simulink model "Waehrungsmodelle"  (R2014a)
settings: Solver=ode1  StartTime=0.0  StopTime=100  FixedStep=1  MaxStep=1  MinStep=1  RelTol=1e-3
(part 12 of 18)

== system Waehrungsmodelle/Währungssystem1/Notenbank ==
  Gesamtkredite : Inport
  Arbeitslosenquote : Inport  Port=2
  Wirtschaftswachtsum : Inport  Port=3
  Inflation : Inport  Port=4
  MATLAB Function : MATLAB Function  TreatAsAtomicUnit=on
  Leitzinssatz der Notenbank : Outport
  Mindestreservesatz von der Notenbank : Outport  Port=2
  Maximale Geldmenge von der Notenbank : Outport  Port=3
  wires:
  MATLAB Function/2(MindestreservesatzOut) -> Mindestreservesatz von der Notenbank/1
  MATLAB Function/3(MaximaleNotenbankGeldmengeOut) -> Maximale Geldmenge von der Notenbank/1
  MATLAB Function/1(LeitzinsOut) -> Leitzinssatz der Notenbank/1
  Wirtschaftswachtsum/1 -> MATLAB Function/4(Wirtschaftswachtsum)
  Arbeitslosenquote/1 -> MATLAB Function/2(Arbeitslosenquote)
  Gesamtkredite/1 -> MATLAB Function/1(Gesamtkredite)
  Inflation/1 -> MATLAB Function/3(Inflation)

== system Waehrungsmodelle/Währungssystem1/Populationsmodell ==
  note: Geburten
  Umweltqualität : Inport
  Dienstleistungsqualität : Inport  Port=2
  Güterangebotsqualität bei vorhandem Einkommen : Inport  Port=3
  Ausgleichsfaktor : Constant  Value=0.3
  Dienstleistungs- multiplikator : Sum
  Divide1 : Product  Inputs=*/
  Divide2 : Product  Inputs=*/
  Divide3 : Product  Inputs=*/
  Erwachsene : Sum  Inputs=+--
  Fertilitätsmultiplikator : Product  Inputs=4
  Fertilitätsrate pro Frau : Constant  Value=3/40
  Frauenanteil pro Erwachsene : Constant  Value=0.5
  Güterangebotsqualitäts- multiplikator : Sum
  Jahre der Altersklasse : Constant  Value=15
  Jahre der Altersklasse1 : Constant  Value=10
  Jahre der Altersklasse2 : Constant  Value=40
  Kinder : Sum  Inputs=+--
  Lebensqualitätsfaktor : Product  Inputs=/
  Product{,1..3} (4 alike) : Product  Inputs=3
  Schüler / Studenten : Sum  Inputs=+--
  Start Erwachsene: 55 : Integrator  InitialCondition=55
  Start Kinder: 13 : Integrator  InitialCondition=13
  Start Schüler: 11 : Integrator  InitialCondition=11
  Sterblichkeitsrate Kinder : Constant  Value=0.003
  Sterblichkeitsrate1 : Constant  Value=0.002
  Sterblichkeitsrate2 : Constant  Value=0.004
  Umwelt- multiplikator : Sum
  Erwerbsfähige : Outport
  wires:
  Product/1 -> Kinder/1
  Jahre der Altersklasse2/1 -> Divide3/2
  Jahre der Altersklasse/1 -> Divide1/2
  Divide1/1 -> Schüler / Studenten/1, Kinder/3
  Sterblichkeitsrate1/1 -> Product1/2
  Sterblichkeitsrate Kinder/1 -> Product2/2
  Divide2/1 -> Schüler / Studenten/3, Erwachsene/1
  Start Schüler: 11/1 -> Product1/3, Divide2/1
  Jahre der Altersklasse1/1 -> Divide2/2
  Sterblichkeitsrate2/1 -> Product3/2
  Start Erwachsene: 55/1 -> Erwerbsfähige/1, Product3/3, Divide3/1, Product/1
  Erwachsene/1 -> Start Erwachsene: 55/1
  Kinder/1 -> Start Kinder: 13/1
  Start Kinder: 13/1 -> Product2/3, Divide1/1
  Schüler / Studenten/1 -> Start Schüler: 11/1
  Ausgleichsfaktor/1 -> Umwelt- multiplikator/2, Güterangebotsqualitäts- multiplikator/1, Dienstleistungs- multiplikator/1
  Fertilitätsmultiplikator/1 -> Product/3
  Umweltqualität/1 -> Umwelt- multiplikator/1
  Dienstleistungs- multiplikator/1 -> Lebensqualitätsfaktor/1, Fertilitätsmultiplikator/4
  Fertilitätsrate pro Frau/1 -> Fertilitätsmultiplikator/1
  Umwelt- multiplikator/1 -> Fertilitätsmultiplikator/2
  Dienstleistungsqualität/1 -> Dienstleistungs- multiplikator/2
  Product2/1 -> Kinder/2
  Product1/1 -> Schüler / Studenten/2
  Divide3/1 -> Erwachsene/3
  Product3/1 -> Erwachsene/2
  Lebensqualitätsfaktor/1 -> Product3/1, Product1/1, Product2/1
  Güterangebotsqualität bei vorhandem Einkommen/1 -> Güterangebotsqualitäts- multiplikator/2
  Güterangebotsqualitäts- multiplikator/1 -> Fertilitätsmultiplikator/3
  Frauenanteil pro Erwachsene/1 -> Product/2

== system Waehrungsmodelle/Währungssystem1/Staat ==
  Kreditvergabe : Inport
  Kreditrückzahlung : Inport  Port=2
  Finanzbedarf Arbeitslosigkeit : Inport  Port=3
  Dienstleistungsqualität : Inport  Port=4
  Steuern Bank : Inport  Port=5
  Steuern Unternehmen : Inport  Port=6
  Rohstoffabgabe : Inport  Port=7
  Umweltqualität : Inport  Port=8
  MATLAB Function : MATLAB Function  TreatAsAtomicUnit=on
  Kreditbedarf : Outport
  Finanzierung Öffentlicher Dienstleistungen : Outport  Port=2
  Geldbestand Staat : Outport  Port=3
  Steuersatz : Outport  Port=4
  Ressourcen Steuer : Outport  Port=5
  wires:
  Steuern Unternehmen/1 -> MATLAB Function/6(SteuernUnternehmen)
  Dienstleistungsqualität/1 -> MATLAB Function/4(Dienstleistungsqualitaet)
  MATLAB Function/4(SteuersatzOut) -> Steuersatz/1
  MATLAB Function/2(FinanzierungOeffentlicheDienstleistungen) -> Finanzierung Öffentlicher Dienstleistungen/1
  Finanzbedarf Arbeitslosigkeit/1 -> MATLAB Function/3(FinanzbedarfArbeitslosigkeit)
  MATLAB Function/3(GeldbestandStaat) -> Geldbestand Staat/1
  Kreditrückzahlung/1 -> MATLAB Function/2(Kreditrueckzahlung)
  MATLAB Function/1(Kreditbedarf) -> Kreditbedarf/1
  Steuern Bank/1 -> MATLAB Function/5(SteuernBanken)
  Kreditvergabe/1 -> MATLAB Function/1(KreditvergabeNeuStaat)
  MATLAB Function/5(RessourcenAbgabesatzOut) -> Ressourcen Steuer/1
  Rohstoffabgabe/1 -> MATLAB Function/7(Rohstoffabgabe)
  Umweltqualität/1 -> MATLAB Function/8(Umweltqualitaet)

== system Waehrungsmodelle/Währungssystem1/Umwelt ==
  Ressourcenbedarf : Inport
  Umwelt : MATLAB Function  TreatAsAtomicUnit=on
  abgebaute Ressourcen : Outport
  verhandene Ressourcen : Outport  Port=2
  Umweltqualität : Outport  Port=3
  wires:
  Umwelt/3(Umweltqualitaet) -> Umweltqualität/1
  Umwelt/2(VorhandeneRessourcenOut) -> verhandene Ressourcen/1
  Umwelt/1(AbgebauteRessourcen) -> abgebaute Ressourcen/1
  Ressourcenbedarf/1 -> Umwelt/1(Ressourcenbedarf)

== system Waehrungsmodelle/Währungssystem1/Unternehmen ==
  Erwerbsfähige : Inport
  Neue Kreditvergabe der Unternehmen : Inport  Port=2
  Kreditrückzahlung der Unternehmen : Inport  Port=3
  Rohstoffe : Inport  Port=4
  Güterkonsum Inland : Inport  Port=5
  Güterkonsum Ausland : Inport  Port=6
  RessourcenAbgabe Steuersatz : Inport  Port=7
  Kreditzinssatz Inland : Inport  Port=8
  Kreditzinssatz Ausland : Inport  Port=9
  Steuersatz : Inport  Port=10
  Neue Kreditvergabe der Unternehmen Ausland : Inport  Port=11
  Kreditrückzahlung der Unternehmen Ausland : Inport  Port=12
  MATLAB Function : MATLAB Function  TreatAsAtomicUnit=on
  Inflation : Outport
  Rohstoffbedarf : Outport  Port=2
  Arbeitsplätze der Unternehmen : Outport  Port=3
  Güterangebot Inland : Outport  Port=4
  Arbeitslohn : Outport  Port=5
  zukünftiger Arbeitsdarf der Unternehmen : Outport  Port=6
  Güterpreis : Outport  Port=7
  Steuern von Unternehmen : Outport  Port=8
  Rohstoffabgabe : Outport  Port=9
  Kreditbedarf Inland : Outport  Port=10
  Kreditbedarf Ausland : Outport  Port=11
  Technischer Fortschritt Rationalität : Outport  Port=12
  Technischer Fortschritt Ressourcen : Outport  Port=13
  Wirtschaftswachstum : Outport  Port=14
  Güterangebot Ausland : Outport  Port=15
  wires:
  MATLAB Function/8(SteuernUnternehmen) -> Steuern von Unternehmen/1
  MATLAB Function/7(GueterpreisOut) -> Güterpreis/1
  Neue Kreditvergabe der Unternehmen/1 -> MATLAB Function/2(NeueKreditvergabeUnternehmen)
  Kreditrückzahlung der Unternehmen/1 -> MATLAB Function/3(KreditrueckzahlungUnternehmen)
  MATLAB Function/6(BenoetigterArbeitsbedarfUnternehmen) -> zukünftiger Arbeitsdarf der Unternehmen/1
  MATLAB Function/4(GueterangebotInland) -> Güterangebot Inland/1
  MATLAB Function/5(ArbeitslohnOut) -> Arbeitslohn/1
  MATLAB Function/2(Rohstoffbedarf) -> Rohstoffbedarf/1
  MATLAB Function/1(Inflation) -> Inflation/1
  Erwerbsfähige/1 -> MATLAB Function/1(Erwerbsfaehige)
  MATLAB Function/3(ArbeitsplaetzeUnternehmen) -> Arbeitsplätze der Unternehmen/1
  Rohstoffe/1 -> MATLAB Function/4(Rohstoffe)
  Güterkonsum Inland/1 -> MATLAB Function/5(GueterkonsumInland)
  MATLAB Function/9(RessourcenAbgabeSteuer) -> Rohstoffabgabe/1
  MATLAB Function/11(KreditbedarfAusland) -> Kreditbedarf Ausland/1
  MATLAB Function/12(TechnischeVerbesserungRationalitaetOut) -> Technischer Fortschritt Rationalität/1
  MATLAB Function/13(TechnischeVerbesserungRessourcenOut) -> Technischer Fortschritt Ressourcen/1
  Güterkonsum Ausland/1 -> MATLAB Function/6(GueterkonsumAusland)
  RessourcenAbgabe Steuersatz/1 -> MATLAB Function/7(RessourcenAbgabeSteuersatz)
  Kreditzinssatz Inland/1 -> MATLAB Function/8(KreditZinssatzInland)
  Kreditzinssatz Ausland/1 -> MATLAB Function/9(KreditZinssatzAusland)
  Steuersatz/1 -> MATLAB Function/10(Steuersatz)
  MATLAB Function/10(KreditbedarfInland) -> Kreditbedarf Inland/1
  MATLAB Function/14(Wirtschaftswachstum) -> Wirtschaftswachstum/1
  MATLAB Function/15(GueterangebotAusland) -> Güterangebot Ausland/1
  Neue Kreditvergabe der Unternehmen Ausland/1 -> MATLAB Function/11(NeueKreditvergabeUnternehmenAusland)
  Kreditrückzahlung der Unternehmen Ausland/1 -> MATLAB Function/12(KreditrueckzahlungUnternehmenAusland)

== system Waehrungsmodelle/Währungssystem1/Wechselkursberechnung ==
  Güterpreis Ausland : Inport
  Güterkonsum im Inland von Gütern vom Ausland : Inport  Port=2
  Güterkonsum im Ausland von Gütern im Inland : Inport  Port=3
  MATLAB Function : MATLAB Function  TreatAsAtomicUnit=on
  Güterpreis Ausland in Eigenwährung : Outport
  Wechselkursfaktor : Outport  Port=2
  Gesamter Güterkonsum im Ausland von Gütern im Inland : Outport  Port=3
  Gesamter Güterkonsum im Inland von Gütern vom Ausland : Outport  Port=4
  wires:
  Güterpreis Ausland/1 -> MATLAB Function/1(GueterpreisAusland)
  Güterkonsum im Inland von Gütern vom Ausland/1 -> MATLAB Function/2(GueterKonsumImInlandVomAusland)
  Güterkonsum im Ausland von Gütern im Inland/1 -> MATLAB Function/3(GueterKonsumImAuslandVomInland)
  MATLAB Function/1(GueterpreisAuslandInEigenwaehrung) -> Güterpreis Ausland in Eigenwährung/1
  MATLAB Function/2(Wechselkursfaktor) -> Wechselkursfaktor/1
  MATLAB Function/3(GesamterGueterKonsumImAuslandVomInlandOut) -> Gesamter Güterkonsum im Ausland von Gütern im Inland/1
  MATLAB Function/4(GesamterGueterKonsumImInlandVomAuslandOut) -> Gesamter Güterkonsum im Inland von Gütern vom Ausland/1

== system Waehrungsmodelle/Währungssystem1/Öffentliche Dienstleistungen ==
  Finanzierung : Inport
  Erwerbsfähige : Inport  Port=2
  Arbeitslohn : Inport  Port=3
  MATLAB Function : MATLAB Function  TreatAsAtomicUnit=on
  Arbeitsplätze Dienstleistung : Outport
  Dienstleistungsqualität : Outport  Port=2
  wires:
  Arbeitslohn/1 -> MATLAB Function/3(Arbeitslohn)
  Erwerbsfähige/1 -> MATLAB Function/2(Erwerbsfaehige)
  Finanzierung/1 -> MATLAB Function/1(Finanzierung)
  MATLAB Function/1(ArbeitsplaetzeDienstleistung) -> Arbeitsplätze Dienstleistung/1
  MATLAB Function/2(Dienstleistungsqualitaet) -> Dienstleistungsqualität/1

== system Waehrungsmodelle/Währungssystem2/Banken ==
  Einlangenänderung der Haushalte : Inport
  Kreditbedarf der Haushalte : Inport  Port=2
  Kreditbedarf der Unternehmen : Inport  Port=3
  Kreditbedarf der Haushalte im Ausland : Inport  Port=4
  Kreditbedarf der Unternehmen im Ausland : Inport  Port=5
  Kreditbedarf des Staates : Inport  Port=6
  Steuersatz : Inport  Port=7
  Leitzins der Notenbank : Inport  Port=8
  Mindestreservesatz der Notenbank : Inport  Port=9
  Maximale Geldmenge der Notebank : Inport  Port=10
  MATLAB Function : MATLAB Function  TreatAsAtomicUnit=on
  Kontostand der Haushalte : Outport
  Kredite der Haushalte : Outport  Port=2
  Kredite der Unternehmen : Outport  Port=3
  Kredite des Staates : Outport  Port=4
  Neue Kreditvergabe Haushalte : Outport  Port=5
  Neue Kreditvergabe Unternehmen : Outport  Port=6
  Neue Kreditvergabe Staat : Outport  Port=7
  Bankgewinn nach Steuern : Outport  Port=8
  Banksteuern : Outport  Port=9
  Bankkontostand : Outport  Port=10
  Bankenzinssatz : Outport  Port=11
  Kreditrückzahlung Staat : Outport  Port=12
  Kreditrückzahlung Haushalte : Outport  Port=13
  Kreditrückzahlung Unternehmen : Outport  Port=14
  Kredite der Unternehmen im Ausland : Outport  Port=15
  Kreditrückzahlung der Unternehmen im Ausland : Outport  Port=16
  Kreditvergabe der Unternehmen im Ausland : Outport  Port=17
  Kredite der Haushalte im Ausland : Outport  Port=18
  Kreditrückzahlung der Haushalte im Ausland : Outport  Port=19
  Kreditvergabe der Haushalte im Ausland : Outport  Port=20
  wires:
  MATLAB Function/1(KontoHaushalteOut) -> Kontostand der Haushalte/1
  MATLAB Function/2(KrediteHaushalteOut) -> Kredite der Haushalte/1
  MATLAB Function/3(KrediteUnternehmenOut) -> Kredite der Unternehmen/1
  MATLAB Function/4(KrediteStaatOut) -> Kredite des Staates/1
  MATLAB Function/5(KreditvergabeHaushalte) -> Neue Kreditvergabe Haushalte/1
  MATLAB Function/6(KreditvergabeUnternehmen) -> Neue Kreditvergabe Unternehmen/1
  MATLAB Function/7(KreditvergabeStaat) -> Neue Kreditvergabe Staat/1
  MATLAB Function/11(BankgewinnNachSteuern) -> Bankgewinn nach Steuern/1
  MATLAB Function/10(KreditrueckzahlungStaat) -> Kreditrückzahlung Staat/1
  MATLAB Function/9(KreditrueckzahlungUnternehmen) -> Kreditrückzahlung Unternehmen/1
  MATLAB Function/8(KreditrueckzahlungHaushalte) -> Kreditrückzahlung Haushalte/1
  MATLAB Function/14(Bankenzinssatz) -> Bankenzinssatz/1
  MATLAB Function/13(BankKontostand) -> Bankkontostand/1
  MATLAB Function/12(BankenSteuern) -> Banksteuern/1
  MATLAB Function/15(KrediteUnternehmenAuslandOut) -> Kredite der Unternehmen im Ausland/1
  MATLAB Function/16(KreditrueckzahlungUnternehmenAusland) -> Kreditrückzahlung der Unternehmen im Ausland/1
  MATLAB Function/17(KreditvergabeUnternehmenAusland) -> Kreditvergabe der Unternehmen im Ausland/1
  MATLAB Function/18(KrediteHaushalteAuslandOut) -> Kredite der Haushalte im Ausland/1
  MATLAB Function/20(KreditvergabeHaushalteAusland) -> Kreditvergabe der Haushalte im Ausland/1
  MATLAB Function/19(KreditrueckzahlungHaushalteAusland) -> Kreditrückzahlung der Haushalte im Ausland/1
  Einlangenänderung der Haushalte/1 -> MATLAB Function/1(EinlagenAenderungHaushalte)
  Kreditbedarf der Haushalte/1 -> MATLAB Function/2(KreditbedarfHaushalte)
  Kreditbedarf der Unternehmen/1 -> MATLAB Function/3(KreditbedarfUnternehmen)
  Kreditbedarf der Haushalte im Ausland/1 -> MATLAB Function/4(KreditbedarfHaushalteAusland)
  Kreditbedarf der Unternehmen im Ausland/1 -> MATLAB Function/5(KreditbedarfUnternehmenAusland)
  Kreditbedarf des Staates/1 -> MATLAB Function/6(KreditbedarfStaat)
  Steuersatz/1 -> MATLAB Function/7(Steuersatz)
  Leitzins der Notenbank/1 -> MATLAB Function/8(Leitzins)
  Mindestreservesatz der Notenbank/1 -> MATLAB Function/9(Mindestreservesatz)
  Maximale Geldmenge der Notebank/1 -> MATLAB Function/10(MaximaleNotenbankGeldmenge)

== system Waehrungsmodelle/Währungssystem2/Haushalte ==
  Erwerbsfähige : Inport
  Arbeitsplätze Dienstleistungen : Inport  Port=2
  Güterangebot Inland : Inport  Port=3
  Arbeitslohn : Inport  Port=4
  Güterpreis Inland : Inport  Port=5
  Neue Kreditvergabe Inland : Inport  Port=6
  Arbeitsplätze Unternehmen : Inport  Port=7
  Kreditrückzahlung Ausland : Inport  Port=8
  Güterpreis Ausland : Inport  Port=9
  Neue Kreditvergabe Ausland : Inport  Port=10
  Kreditrückzahlung Inland : Inport  Port=11
  Güterangebot Ausland : Inport  Port=12
  Kreditzinssatz Inland : Inport  Port=13
  Kreditzinssatz Ausland : Inport  Port=14
  MATLAB Function : MATLAB Function  TreatAsAtomicUnit=on
  Güterkonsum Inland : Outport
  Finanzbedarf Arbeitslosigkeit : Outport  Port=2
  Spareinlagen : Outport  Port=3
  Kreditbedarf Inland : Outport  Port=4
  Arbeiter Unternehmen : Outport  Port=5
  Gütervorrat der Haushalte : Outport  Port=6
  Güterangebotsqualität : Outport  Port=7
  Arbeitslosenquote : Outport  Port=8
  Güterkonsum Ausland : Outport  Port=9
  Kreditbedarf Ausland : Outport  Port=10
  wires:
  Arbeitslohn/1 -> MATLAB Function/7(Arbeitslohn)
  Erwerbsfähige/1 -> MATLAB Function/1(Erwerbsfaehige)
  Arbeitsplätze Dienstleistungen/1 -> MATLAB Function/2(ArbeitsplaetzeDienstleistungen)
  Güterangebot Inland/1 -> MATLAB Function/6(GueterAngebotInland)
  Güterpreis Inland/1 -> MATLAB Function/8(GueterpreisInland)
  MATLAB Function/1(GueterkonsumInland) -> Güterkonsum Inland/1
  MATLAB Function/2(FinanzierungArbeitslosigkeit) -> Finanzbedarf Arbeitslosigkeit/1
  MATLAB Function/4(KreditbedarfInland) -> Kreditbedarf Inland/1
  MATLAB Function/5(ArbeiterUnternehmen) -> Arbeiter Unternehmen/1
  MATLAB Function/3(Spareinlagen) -> Spareinlagen/1
  Neue Kreditvergabe Inland/1 -> MATLAB Function/4(NeueKreditvergabeInland)
  Arbeitsplätze Unternehmen/1 -> MATLAB Function/3(ArbeitsplaetzeUnternehmen)
  MATLAB Function/6(GueterVorratHaushalte) -> Gütervorrat der Haushalte/1
  MATLAB Function/7(GueterangebotsqualitaetOut) -> Güterangebotsqualität/1
  Kreditrückzahlung Ausland/1 -> MATLAB Function/5(KreditrueckzahlungInland)
  MATLAB Function/8(Arbeitslosenquote) -> Arbeitslosenquote/1
  MATLAB Function/9(GueterkonsumAusland) -> Güterkonsum Ausland/1
  MATLAB Function/10(KreditbedarfAusland) -> Kreditbedarf Ausland/1
  Güterpreis Ausland/1 -> MATLAB Function/9(GueterpreisAusland)
  Neue Kreditvergabe Ausland/1 -> MATLAB Function/10(NeueKreditvergabeAusland)
  Kreditrückzahlung Inland/1 -> MATLAB Function/11(KreditrueckzahlungAusland)
  Güterangebot Ausland/1 -> MATLAB Function/12(GueterAngebotAusland)
  Kreditzinssatz Inland/1 -> MATLAB Function/13(KreditZinssatzInland)
  Kreditzinssatz Ausland/1 -> MATLAB Function/14(KreditZinssatzAusland)

== system Waehrungsmodelle/Währungssystem2/Notenbank ==
  Gesamtkredite : Inport
  Arbeitslosenquote : Inport  Port=2
  Wirtschaftswachtsum : Inport  Port=3
  Inflation : Inport  Port=4
  MATLAB Function : MATLAB Function  TreatAsAtomicUnit=on
  Leitzinssatz der Notenbank : Outport
  Mindestreservesatz von der Notenbank : Outport  Port=2
  Maximale Geldmenge von der Notenbank : Outport  Port=3
  wires:
  MATLAB Function/2(MindestreservesatzOut) -> Mindestreservesatz von der Notenbank/1
  MATLAB Function/3(MaximaleNotenbankGeldmengeOut) -> Maximale Geldmenge von der Notenbank/1
  MATLAB Function/1(LeitzinsOut) -> Leitzinssatz der Notenbank/1
  Wirtschaftswachtsum/1 -> MATLAB Function/4(Wirtschaftswachtsum)
  Arbeitslosenquote/1 -> MATLAB Function/2(Arbeitslosenquote)
  Gesamtkredite/1 -> MATLAB Function/1(Gesamtkredite)
  Inflation/1 -> MATLAB Function/3(Inflation)

== system Waehrungsmodelle/Währungssystem2/Populationsmodell ==
  note: Geburten
  Umweltqualität : Inport
  Dienstleistungsqualität : Inport  Port=2
  Güterangebotsqualität bei vorhandem Einkommen : Inport  Port=3
  Ausgleichsfaktor : Constant  Value=0.3
  Dienstleistungs- multiplikator : Sum
  Divide1 : Product  Inputs=*/
  Divide2 : Product  Inputs=*/
  Divide3 : Product  Inputs=*/
  Erwachsene : Sum  Inputs=+--
  Fertilitätsmultiplikator : Product  Inputs=4
  Fertilitätsrate pro Frau : Constant  Value=3/40
  Frauenanteil pro Erwachsene : Constant  Value=0.5
  Güterangebotsqualitäts- multiplikator : Sum
  Jahre der Altersklasse : Constant  Value=15
  Jahre der Altersklasse1 : Constant  Value=10
  Jahre der Altersklasse2 : Constant  Value=40
  Kinder : Sum  Inputs=+--
  Lebensqualitätsfaktor : Product  Inputs=/
  Product{,1..3} (4 alike) : Product  Inputs=3
  Schüler / Studenten : Sum  Inputs=+--
  Start Erwachsene: 55 : Integrator  InitialCondition=55
  Start Kinder: 13 : Integrator  InitialCondition=13
  Start Schüler: 11 : Integrator  InitialCondition=11
  Sterblichkeitsrate Kinder : Constant  Value=0.003
  Sterblichkeitsrate1 : Constant  Value=0.002
  Sterblichkeitsrate2 : Constant  Value=0.004
  Umwelt- multiplikator : Sum
  Erwerbsfähige : Outport
  wires:
  Product/1 -> Kinder/1
  Jahre der Altersklasse2/1 -> Divide3/2
  Jahre der Altersklasse/1 -> Divide1/2
  Divide1/1 -> Schüler / Studenten/1, Kinder/3
  Sterblichkeitsrate1/1 -> Product1/2
  Sterblichkeitsrate Kinder/1 -> Product2/2
  Divide2/1 -> Schüler / Studenten/3, Erwachsene/1
  Start Schüler: 11/1 -> Product1/3, Divide2/1
  Jahre der Altersklasse1/1 -> Divide2/2
  Sterblichkeitsrate2/1 -> Product3/2
  Start Erwachsene: 55/1 -> Erwerbsfähige/1, Product3/3, Divide3/1, Product/1
  Erwachsene/1 -> Start Erwachsene: 55/1
  Kinder/1 -> Start Kinder: 13/1
  Start Kinder: 13/1 -> Product2/3, Divide1/1
  Schüler / Studenten/1 -> Start Schüler: 11/1
  Ausgleichsfaktor/1 -> Umwelt- multiplikator/2, Güterangebotsqualitäts- multiplikator/1, Dienstleistungs- multiplikator/1
  Fertilitätsmultiplikator/1 -> Product/3
  Umweltqualität/1 -> Umwelt- multiplikator/1
  Dienstleistungs- multiplikator/1 -> Lebensqualitätsfaktor/1, Fertilitätsmultiplikator/4
  Fertilitätsrate pro Frau/1 -> Fertilitätsmultiplikator/1
  Umwelt- multiplikator/1 -> Fertilitätsmultiplikator/2
  Dienstleistungsqualität/1 -> Dienstleistungs- multiplikator/2
  Product2/1 -> Kinder/2
  Product1/1 -> Schüler / Studenten/2
  Divide3/1 -> Erwachsene/3
  Product3/1 -> Erwachsene/2
  Lebensqualitätsfaktor/1 -> Product3/1, Product1/1, Product2/1
  Güterangebotsqualität bei vorhandem Einkommen/1 -> Güterangebotsqualitäts- multiplikator/2
  Güterangebotsqualitäts- multiplikator/1 -> Fertilitätsmultiplikator/3
  Frauenanteil pro Erwachsene/1 -> Product/2

== system Waehrungsmodelle/Währungssystem2/Staat ==
  Kreditvergabe : Inport
  Kreditrückzahlung : Inport  Port=2
  Finanzbedarf Arbeitslosigkeit : Inport  Port=3
  Dienstleistungsqualität : Inport  Port=4
  Steuern Bank : Inport  Port=5
  Steuern Unternehmen : Inport  Port=6
  Rohstoffabgabe : Inport  Port=7
  Umweltqualität : Inport  Port=8
  MATLAB Function : MATLAB Function  TreatAsAtomicUnit=on
  Kreditbedarf : Outport
  Finanzierung Öffentlicher Dienstleistungen : Outport  Port=2
  Geldbestand Staat : Outport  Port=3
  Steuersatz : Outport  Port=4
  Ressourcen Steuer : Outport  Port=5
  wires:
  Steuern Unternehmen/1 -> MATLAB Function/6(SteuernUnternehmen)
  Dienstleistungsqualität/1 -> MATLAB Function/4(Dienstleistungsqualitaet)
  MATLAB Function/4(SteuersatzOut) -> Steuersatz/1
  MATLAB Function/2(FinanzierungOeffentlicheDienstleistungen) -> Finanzierung Öffentlicher Dienstleistungen/1
  Finanzbedarf Arbeitslosigkeit/1 -> MATLAB Function/3(FinanzbedarfArbeitslosigkeit)
  MATLAB Function/3(GeldbestandStaat) -> Geldbestand Staat/1
  Kreditrückzahlung/1 -> MATLAB Function/2(Kreditrueckzahlung)
  MATLAB Function/1(Kreditbedarf) -> Kreditbedarf/1
  Steuern Bank/1 -> MATLAB Function/5(SteuernBanken)
  Kreditvergabe/1 -> MATLAB Function/1(KreditvergabeNeuStaat)
  MATLAB Function/5(RessourcenAbgabesatzOut) -> Ressourcen Steuer/1
  Rohstoffabgabe/1 -> MATLAB Function/7(Rohstoffabgabe)
  Umweltqualität/1 -> MATLAB Function/8(Umweltqualitaet)

== system Waehrungsmodelle/Währungssystem2/Umwelt ==
  Ressourcenbedarf : Inport
  Umwelt : MATLAB Function  TreatAsAtomicUnit=on
  abgebaute Ressourcen : Outport
  verhandene Ressourcen : Outport  Port=2
  Umweltqualität : Outport  Port=3
  wires:
  Umwelt/3(Umweltqualitaet) -> Umweltqualität/1
  Umwelt/2(VorhandeneRessourcenOut) -> verhandene Ressourcen/1
  Umwelt/1(AbgebauteRessourcen) -> abgebaute Ressourcen/1
  Ressourcenbedarf/1 -> Umwelt/1(Ressourcenbedarf)

== system Waehrungsmodelle/Währungssystem2/Unternehmen ==
  Erwerbsfähige : Inport
  Neue Kreditvergabe der Unternehmen : Inport  Port=2
  Kreditrückzahlung der Unternehmen : Inport  Port=3
  Rohstoffe : Inport  Port=4
  Güterkonsum Inland : Inport  Port=5
  Güterkonsum Ausland : Inport  Port=6
  RessourcenAbgabe Steuersatz : Inport  Port=7
  Kreditzinssatz Inland : Inport  Port=8
  Kreditzinssatz Ausland : Inport  Port=9
  Steuersatz : Inport  Port=10
  Neue Kreditvergabe der Unternehmen Ausland : Inport  Port=11
  Kreditrückzahlung der Unternehmen Ausland : Inport  Port=12
  MATLAB Function : MATLAB Function  TreatAsAtomicUnit=on
  Inflation : Outport
  Rohstoffbedarf : Outport  Port=2
  Arbeitsplätze der Unternehmen : Outport  Port=3
  Güterangebot Inland : Outport  Port=4
  Arbeitslohn : Outport  Port=5
  zukünftiger Arbeitsdarf der Unternehmen : Outport  Port=6
  Güterpreis : Outport  Port=7
  Steuern von Unternehmen : Outport  Port=8
  Rohstoffabgabe : Outport  Port=9
  Kreditbedarf Inland : Outport  Port=10
  Kreditbedarf Ausland : Outport  Port=11
  Technischer Fortschritt Rationalität : Outport  Port=12
  Technischer Fortschritt Ressourcen : Outport  Port=13
  Wirtschaftswachstum : Outport  Port=14
  Güterangebot Ausland : Outport  Port=15
  wires:
  MATLAB Function/8(SteuernUnternehmen) -> Steuern von Unternehmen/1
  MATLAB Function/7(GueterpreisOut) -> Güterpreis/1
  Neue Kreditvergabe der Unternehmen/1 -> MATLAB Function/2(NeueKreditvergabeUnternehmen)
  Kreditrückzahlung der Unternehmen/1 -> MATLAB Function/3(KreditrueckzahlungUnternehmen)
  MATLAB Function/6(BenoetigterArbeitsbedarfUnternehmen) -> zukünftiger Arbeitsdarf der Unternehmen/1
  MATLAB Function/4(GueterangebotInland) -> Güterangebot Inland/1
  MATLAB Function/5(ArbeitslohnOut) -> Arbeitslohn/1
  MATLAB Function/2(Rohstoffbedarf) -> Rohstoffbedarf/1
  MATLAB Function/1(Inflation) -> Inflation/1
  Erwerbsfähige/1 -> MATLAB Function/1(Erwerbsfaehige)
  MATLAB Function/3(ArbeitsplaetzeUnternehmen) -> Arbeitsplätze der Unternehmen/1
  Rohstoffe/1 -> MATLAB Function/4(Rohstoffe)
  Güterkonsum Inland/1 -> MATLAB Function/5(GueterkonsumInland)
  MATLAB Function/9(RessourcenAbgabeSteuer) -> Rohstoffabgabe/1
  MATLAB Function/11(KreditbedarfAusland) -> Kreditbedarf Ausland/1
  MATLAB Function/12(TechnischeVerbesserungRationalitaetOut) -> Technischer Fortschritt Rationalität/1
  MATLAB Function/13(TechnischeVerbesserungRessourcenOut) -> Technischer Fortschritt Ressourcen/1
  Güterkonsum Ausland/1 -> MATLAB Function/6(GueterkonsumAusland)
  RessourcenAbgabe Steuersatz/1 -> MATLAB Function/7(RessourcenAbgabeSteuersatz)
  Kreditzinssatz Inland/1 -> MATLAB Function/8(KreditZinssatzInland)
  Kreditzinssatz Ausland/1 -> MATLAB Function/9(KreditZinssatzAusland)
  Steuersatz/1 -> MATLAB Function/10(Steuersatz)
  MATLAB Function/10(KreditbedarfInland) -> Kreditbedarf Inland/1
  MATLAB Function/14(Wirtschaftswachstum) -> Wirtschaftswachstum/1
  MATLAB Function/15(GueterangebotAusland) -> Güterangebot Ausland/1
  Neue Kreditvergabe der Unternehmen Ausland/1 -> MATLAB Function/11(NeueKreditvergabeUnternehmenAusland)
  Kreditrückzahlung der Unternehmen Ausland/1 -> MATLAB Function/12(KreditrueckzahlungUnternehmenAusland)

== system Waehrungsmodelle/Währungssystem2/Wechselkursberechnung ==
  Güterpreis Ausland : Inport
  Güterkonsum im Inland von Gütern vom Ausland : Inport  Port=2
  Güterkonsum im Ausland von Gütern im Inland : Inport  Port=3
  MATLAB Function : MATLAB Function  TreatAsAtomicUnit=on
  Güterpreis Ausland in Eigenwährung : Outport
  Wechselkursfaktor : Outport  Port=2
  Gesamter Güterkonsum im Ausland von Gütern im Inland : Outport  Port=3
  Gesamter Güterkonsum im Inland von Gütern vom Ausland : Outport  Port=4
  wires:
  Güterpreis Ausland/1 -> MATLAB Function/1(GueterpreisAusland)
  Güterkonsum im Inland von Gütern vom Ausland/1 -> MATLAB Function/2(GueterKonsumImInlandVomAusland)
  Güterkonsum im Ausland von Gütern im Inland/1 -> MATLAB Function/3(GueterKonsumImAuslandVomInland)
  MATLAB Function/1(GueterpreisAuslandInEigenwaehrung) -> Güterpreis Ausland in Eigenwährung/1
  MATLAB Function/2(Wechselkursfaktor) -> Wechselkursfaktor/1
  MATLAB Function/3(GesamterGueterKonsumImAuslandVomInlandOut) -> Gesamter Güterkonsum im Ausland von Gütern im Inland/1
  MATLAB Function/4(GesamterGueterKonsumImInlandVomAuslandOut) -> Gesamter Güterkonsum im Inland von Gütern vom Ausland/1

== system Waehrungsmodelle/Währungssystem2/Öffentliche Dienstleistungen ==
  Finanzierung : Inport
  Erwerbsfähige : Inport  Port=2
  Arbeitslohn : Inport  Port=3
  MATLAB Function : MATLAB Function  TreatAsAtomicUnit=on
  Arbeitsplätze Dienstleistung : Outport
  Dienstleistungsqualität : Outport  Port=2
  wires:
  Arbeitslohn/1 -> MATLAB Function/3(Arbeitslohn)
  Erwerbsfähige/1 -> MATLAB Function/2(Erwerbsfaehige)
  Finanzierung/1 -> MATLAB Function/1(Finanzierung)
  MATLAB Function/1(ArbeitsplaetzeDienstleistung) -> Arbeitsplätze Dienstleistung/1
  MATLAB Function/2(Dienstleistungsqualitaet) -> Dienstleistungsqualität/1

== system Waehrungsmodelle/Währungssystem3/Banken ==
  Einlangenänderung der Haushalte : Inport
  Kreditbedarf der Haushalte : Inport  Port=2
  Kreditbedarf der Unternehmen : Inport  Port=3
  Kreditbedarf der Haushalte im Ausland : Inport  Port=4
  Kreditbedarf der Unternehmen im Ausland : Inport  Port=5
  Kreditbedarf des Staates : Inport  Port=6
  Steuersatz : Inport  Port=7
  Leitzins der Notenbank : Inport  Port=8
  Mindestreservesatz der Notenbank : Inport  Port=9
  Maximale Geldmenge der Notebank : Inport  Port=10
  MATLAB Function : MATLAB Function  TreatAsAtomicUnit=on
  Kontostand der Haushalte : Outport
  Kredite der Haushalte : Outport  Port=2
  Kredite der Unternehmen : Outport  Port=3
  Kredite des Staates : Outport  Port=4
  Neue Kreditvergabe Haushalte : Outport  Port=5
  Neue Kreditvergabe Unternehmen : Outport  Port=6
  Neue Kreditvergabe Staat : Outport  Port=7
  Bankgewinn nach Steuern : Outport  Port=8
  Banksteuern : Outport  Port=9
  Bankkontostand : Outport  Port=10
  Bankenzinssatz : Outport  Port=11
  Kreditrückzahlung Staat : Outport  Port=12
  Kreditrückzahlung Haushalte : Outport  Port=13
  Kreditrückzahlung Unternehmen : Outport  Port=14
  Kredite der Unternehmen im Ausland : Outport  Port=15
  Kreditrückzahlung der Unternehmen im Ausland : Outport  Port=16
  Kreditvergabe der Unternehmen im Ausland : Outport  Port=17
  Kredite der Haushalte im Ausland : Outport  Port=18
  Kreditrückzahlung der Haushalte im Ausland : Outport  Port=19
  Kreditvergabe der Haushalte im Ausland : Outport  Port=20
  wires:
  MATLAB Function/1(KontoHaushalteOut) -> Kontostand der Haushalte/1
  MATLAB Function/2(KrediteHaushalteOut) -> Kredite der Haushalte/1
  MATLAB Function/3(KrediteUnternehmenOut) -> Kredite der Unternehmen/1
  MATLAB Function/4(KrediteStaatOut) -> Kredite des Staates/1
  MATLAB Function/5(KreditvergabeHaushalte) -> Neue Kreditvergabe Haushalte/1
  MATLAB Function/6(KreditvergabeUnternehmen) -> Neue Kreditvergabe Unternehmen/1
  MATLAB Function/7(KreditvergabeStaat) -> Neue Kreditvergabe Staat/1
  MATLAB Function/11(BankgewinnNachSteuern) -> Bankgewinn nach Steuern/1
  MATLAB Function/10(KreditrueckzahlungStaat) -> Kreditrückzahlung Staat/1
  MATLAB Function/9(KreditrueckzahlungUnternehmen) -> Kreditrückzahlung Unternehmen/1
  MATLAB Function/8(KreditrueckzahlungHaushalte) -> Kreditrückzahlung Haushalte/1
  MATLAB Function/14(Bankenzinssatz) -> Bankenzinssatz/1
  MATLAB Function/13(BankKontostand) -> Bankkontostand/1
  MATLAB Function/12(BankenSteuern) -> Banksteuern/1
  MATLAB Function/15(KrediteUnternehmenAuslandOut) -> Kredite der Unternehmen im Ausland/1
  MATLAB Function/16(KreditrueckzahlungUnternehmenAusland) -> Kreditrückzahlung der Unternehmen im Ausland/1
  MATLAB Function/17(KreditvergabeUnternehmenAusland) -> Kreditvergabe der Unternehmen im Ausland/1
  MATLAB Function/18(KrediteHaushalteAuslandOut) -> Kredite der Haushalte im Ausland/1
  MATLAB Function/20(KreditvergabeHaushalteAusland) -> Kreditvergabe der Haushalte im Ausland/1
  MATLAB Function/19(KreditrueckzahlungHaushalteAusland) -> Kreditrückzahlung der Haushalte im Ausland/1
  Einlangenänderung der Haushalte/1 -> MATLAB Function/1(EinlagenAenderungHaushalte)
  Kreditbedarf der Haushalte/1 -> MATLAB Function/2(KreditbedarfHaushalte)
  Kreditbedarf der Unternehmen/1 -> MATLAB Function/3(KreditbedarfUnternehmen)
  Kreditbedarf der Haushalte im Ausland/1 -> MATLAB Function/4(KreditbedarfHaushalteAusland)
  Kreditbedarf der Unternehmen im Ausland/1 -> MATLAB Function/5(KreditbedarfUnternehmenAusland)
  Kreditbedarf des Staates/1 -> MATLAB Function/6(KreditbedarfStaat)
  Steuersatz/1 -> MATLAB Function/7(Steuersatz)
  Leitzins der Notenbank/1 -> MATLAB Function/8(Leitzins)
  Mindestreservesatz der Notenbank/1 -> MATLAB Function/9(Mindestreservesatz)
  Maximale Geldmenge der Notebank/1 -> MATLAB Function/10(MaximaleNotenbankGeldmenge)

== system Waehrungsmodelle/Währungssystem3/Haushalte ==
  Erwerbsfähige : Inport
  Arbeitsplätze Dienstleistungen : Inport  Port=2
  Güterangebot Inland : Inport  Port=3
  Arbeitslohn : Inport  Port=4
  Güterpreis Inland : Inport  Port=5
  Neue Kreditvergabe Inland : Inport  Port=6
  Arbeitsplätze Unternehmen : Inport  Port=7
  Kreditrückzahlung Ausland : Inport  Port=8
  Güterpreis Ausland : Inport  Port=9
  Neue Kreditvergabe Ausland : Inport  Port=10
  Kreditrückzahlung Inland : Inport  Port=11
  Güterangebot Ausland : Inport  Port=12
  Kreditzinssatz Inland : Inport  Port=13
  Kreditzinssatz Ausland : Inport  Port=14
  MATLAB Function : MATLAB Function  TreatAsAtomicUnit=on
  Güterkonsum Inland : Outport
  Finanzbedarf Arbeitslosigkeit : Outport  Port=2
  Spareinlagen : Outport  Port=3
  Kreditbedarf Inland : Outport  Port=4
  Arbeiter Unternehmen : Outport  Port=5
  Gütervorrat der Haushalte : Outport  Port=6
  Güterangebotsqualität : Outport  Port=7
  Arbeitslosenquote : Outport  Port=8
  Güterkonsum Ausland : Outport  Port=9
  Kreditbedarf Ausland : Outport  Port=10
  wires:
  Arbeitslohn/1 -> MATLAB Function/7(Arbeitslohn)
  Erwerbsfähige/1 -> MATLAB Function/1(Erwerbsfaehige)
  Arbeitsplätze Dienstleistungen/1 -> MATLAB Function/2(ArbeitsplaetzeDienstleistungen)
  Güterangebot Inland/1 -> MATLAB Function/6(GueterAngebotInland)
  Güterpreis Inland/1 -> MATLAB Function/8(GueterpreisInland)
  MATLAB Function/1(GueterkonsumInland) -> Güterkonsum Inland/1
  MATLAB Function/2(FinanzierungArbeitslosigkeit) -> Finanzbedarf Arbeitslosigkeit/1
  MATLAB Function/4(KreditbedarfInland) -> Kreditbedarf Inland/1
  MATLAB Function/5(ArbeiterUnternehmen) -> Arbeiter Unternehmen/1
  MATLAB Function/3(Spareinlagen) -> Spareinlagen/1
  Neue Kreditvergabe Inland/1 -> MATLAB Function/4(NeueKreditvergabeInland)
  Arbeitsplätze Unternehmen/1 -> MATLAB Function/3(ArbeitsplaetzeUnternehmen)
  MATLAB Function/6(GueterVorratHaushalte) -> Gütervorrat der Haushalte/1
  MATLAB Function/7(GueterangebotsqualitaetOut) -> Güterangebotsqualität/1
  Kreditrückzahlung Ausland/1 -> MATLAB Function/5(KreditrueckzahlungInland)
  MATLAB Function/8(Arbeitslosenquote) -> Arbeitslosenquote/1
  MATLAB Function/9(GueterkonsumAusland) -> Güterkonsum Ausland/1
  MATLAB Function/10(KreditbedarfAusland) -> Kreditbedarf Ausland/1
  Güterpreis Ausland/1 -> MATLAB Function/9(GueterpreisAusland)
  Neue Kreditvergabe Ausland/1 -> MATLAB Function/10(NeueKreditvergabeAusland)
  Kreditrückzahlung Inland/1 -> MATLAB Function/11(KreditrueckzahlungAusland)
  Güterangebot Ausland/1 -> MATLAB Function/12(GueterAngebotAusland)
  Kreditzinssatz Inland/1 -> MATLAB Function/13(KreditZinssatzInland)
  Kreditzinssatz Ausland/1 -> MATLAB Function/14(KreditZinssatzAusland)

== system Waehrungsmodelle/Währungssystem3/Notenbank ==
  Gesamtkredite : Inport
  Arbeitslosenquote : Inport  Port=2
  Wirtschaftswachtsum : Inport  Port=3
  Inflation : Inport  Port=4
  MATLAB Function : MATLAB Function  TreatAsAtomicUnit=on
  Leitzinssatz der Notenbank : Outport
  Mindestreservesatz von der Notenbank : Outport  Port=2
  Maximale Geldmenge von der Notenbank : Outport  Port=3
  wires:
  MATLAB Function/2(MindestreservesatzOut) -> Mindestreservesatz von der Notenbank/1
  MATLAB Function/3(MaximaleNotenbankGeldmengeOut) -> Maximale Geldmenge von der Notenbank/1
  MATLAB Function/1(LeitzinsOut) -> Leitzinssatz der Notenbank/1
  Wirtschaftswachtsum/1 -> MATLAB Function/4(Wirtschaftswachtsum)
  Arbeitslosenquote/1 -> MATLAB Function/2(Arbeitslosenquote)
  Gesamtkredite/1 -> MATLAB Function/1(Gesamtkredite)
  Inflation/1 -> MATLAB Function/3(Inflation)

== system Waehrungsmodelle/Währungssystem3/Populationsmodell ==
  note: Geburten
  Umweltqualität : Inport
  Dienstleistungsqualität : Inport  Port=2
  Güterangebotsqualität bei vorhandem Einkommen : Inport  Port=3
  Ausgleichsfaktor : Constant  Value=0.3
  Dienstleistungs- multiplikator : Sum
  Divide1 : Product  Inputs=*/
  Divide2 : Product  Inputs=*/
  Divide3 : Product  Inputs=*/
  Erwachsene : Sum  Inputs=+--
  Fertilitätsmultiplikator : Product  Inputs=4
  Fertilitätsrate pro Frau : Constant  Value=3/40
  Frauenanteil pro Erwachsene : Constant  Value=0.5
  Güterangebotsqualitäts- multiplikator : Sum
  Jahre der Altersklasse : Constant  Value=15
  Jahre der Altersklasse1 : Constant  Value=10
  Jahre der Altersklasse2 : Constant  Value=40
  Kinder : Sum  Inputs=+--
  Lebensqualitätsfaktor : Product  Inputs=/
  Product{,1..3} (4 alike) : Product  Inputs=3
  Schüler / Studenten : Sum  Inputs=+--
  Start Erwachsene: 55 : Integrator  InitialCondition=55
  Start Kinder: 13 : Integrator  InitialCondition=13
  Start Schüler: 11 : Integrator  InitialCondition=11
  Sterblichkeitsrate Kinder : Constant  Value=0.003
  Sterblichkeitsrate1 : Constant  Value=0.002
  Sterblichkeitsrate2 : Constant  Value=0.004
  Umwelt- multiplikator : Sum
  Erwerbsfähige : Outport
  wires:
  Product/1 -> Kinder/1
  Jahre der Altersklasse2/1 -> Divide3/2
  Jahre der Altersklasse/1 -> Divide1/2
  Divide1/1 -> Schüler / Studenten/1, Kinder/3
  Sterblichkeitsrate1/1 -> Product1/2
  Sterblichkeitsrate Kinder/1 -> Product2/2
  Divide2/1 -> Schüler / Studenten/3, Erwachsene/1
  Start Schüler: 11/1 -> Product1/3, Divide2/1
  Jahre der Altersklasse1/1 -> Divide2/2
  Sterblichkeitsrate2/1 -> Product3/2
  Start Erwachsene: 55/1 -> Erwerbsfähige/1, Product3/3, Divide3/1, Product/1
  Erwachsene/1 -> Start Erwachsene: 55/1
  Kinder/1 -> Start Kinder: 13/1
  Start Kinder: 13/1 -> Product2/3, Divide1/1
  Schüler / Studenten/1 -> Start Schüler: 11/1
  Ausgleichsfaktor/1 -> Umwelt- multiplikator/2, Güterangebotsqualitäts- multiplikator/1, Dienstleistungs- multiplikator/1
  Fertilitätsmultiplikator/1 -> Product/3
  Umweltqualität/1 -> Umwelt- multiplikator/1
  Dienstleistungs- multiplikator/1 -> Lebensqualitätsfaktor/1, Fertilitätsmultiplikator/4
  Fertilitätsrate pro Frau/1 -> Fertilitätsmultiplikator/1
  Umwelt- multiplikator/1 -> Fertilitätsmultiplikator/2
  Dienstleistungsqualität/1 -> Dienstleistungs- multiplikator/2
  Product2/1 -> Kinder/2
  Product1/1 -> Schüler / Studenten/2
  Divide3/1 -> Erwachsene/3
  Product3/1 -> Erwachsene/2
  Lebensqualitätsfaktor/1 -> Product3/1, Product1/1, Product2/1
  Güterangebotsqualität bei vorhandem Einkommen/1 -> Güterangebotsqualitäts- multiplikator/2
  Güterangebotsqualitäts- multiplikator/1 -> Fertilitätsmultiplikator/3
  Frauenanteil pro Erwachsene/1 -> Product/2

== system Waehrungsmodelle/Währungssystem3/Staat ==
  Kreditvergabe : Inport
  Kreditrückzahlung : Inport  Port=2
  Finanzbedarf Arbeitslosigkeit : Inport  Port=3
  Dienstleistungsqualität : Inport  Port=4
  Steuern Bank : Inport  Port=5
  Steuern Unternehmen : Inport  Port=6
  Rohstoffabgabe : Inport  Port=7
  Umweltqualität : Inport  Port=8
  MATLAB Function : MATLAB Function  TreatAsAtomicUnit=on
  Kreditbedarf : Outport
  Finanzierung Öffentlicher Dienstleistungen : Outport  Port=2
  Geldbestand Staat : Outport  Port=3
  Steuersatz : Outport  Port=4
  Ressourcen Steuer : Outport  Port=5
  wires:
  Steuern Unternehmen/1 -> MATLAB Function/6(SteuernUnternehmen)
  Dienstleistungsqualität/1 -> MATLAB Function/4(Dienstleistungsqualitaet)
  MATLAB Function/4(SteuersatzOut) -> Steuersatz/1
  MATLAB Function/2(FinanzierungOeffentlicheDienstleistungen) -> Finanzierung Öffentlicher Dienstleistungen/1
  Finanzbedarf Arbeitslosigkeit/1 -> MATLAB Function/3(FinanzbedarfArbeitslosigkeit)
  MATLAB Function/3(GeldbestandStaat) -> Geldbestand Staat/1
  Kreditrückzahlung/1 -> MATLAB Function/2(Kreditrueckzahlung)
  MATLAB Function/1(Kreditbedarf) -> Kreditbedarf/1
  Steuern Bank/1 -> MATLAB Function/5(SteuernBanken)
  Kreditvergabe/1 -> MATLAB Function/1(KreditvergabeNeuStaat)
  MATLAB Function/5(RessourcenAbgabesatzOut) -> Ressourcen Steuer/1
  Rohstoffabgabe/1 -> MATLAB Function/7(Rohstoffabgabe)
  Umweltqualität/1 -> MATLAB Function/8(Umweltqualitaet)

== system Waehrungsmodelle/Währungssystem3/Umwelt ==
  Ressourcenbedarf : Inport
  Umwelt : MATLAB Function  TreatAsAtomicUnit=on
  abgebaute Ressourcen : Outport
  verhandene Ressourcen : Outport  Port=2
  Umweltqualität : Outport  Port=3
  wires:
  Umwelt/3(Umweltqualitaet) -> Umweltqualität/1
  Umwelt/2(VorhandeneRessourcenOut) -> verhandene Ressourcen/1
  Umwelt/1(AbgebauteRessourcen) -> abgebaute Ressourcen/1
  Ressourcenbedarf/1 -> Umwelt/1(Ressourcenbedarf)

== matlab function Waehrungsmodelle/Währungssystem2/Öffentliche Dienstleistungen/MATLAB Function ==
  data: Finanzierung input; ArbeitsplaetzeDienstleistung output; Erwerbsfaehige input; Arbeitslohn input; Dienstleistungsqualitaet output
function [ArbeitsplaetzeDienstleistung, Dienstleistungsqualitaet] = OeffentlicheDienstleistungen(Finanzierung, Erwerbsfaehige, Arbeitslohn)
%# Submodul zur Berechnung das Öffentliche Dienstleistungsmodell

    persistent Arbeitsplaetze;

    % Anfangsarbeitsplätze
    if isempty(Arbeitsplaetze)
       Arbeitsplaetze = 20;
    end 

    % Da der Arbeitslohn ein Referenzlohn der privaten Unternehmen ist wird
    % dieser angepasst und um 20 % gesenkt
    LohnNiveauOeffentlicherDienst = 0.8;
    Arbeitslohn = Arbeitslohn * LohnNiveauOeffentlicherDienst;
    
    % Es können nicht mehr Arbeitsplätze wie Erwerbsfähige vorhanden sind
    % besetzt werden
    if Erwerbsfaehige < Arbeitsplaetze
        Arbeitsplaetze = Erwerbsfaehige;
    end

    % Existiert nicht genug Geld für die öffentlichen Dientleistungen
    % werden die Arbeitsplätze an die Finanzierung vom Staat angepasst.
    if (Finanzierung < Arbeitsplaetze * Arbeitslohn)
        Arbeitsplaetze = floor(Finanzierung / Arbeitslohn);        
    end          
       
    ArbeitsplaetzeDienstleistung = Arbeitsplaetze;
    
    % Berechnet Dienstleistungsqualitaet mit min:0.2 und max:1
    % indem die Arbeitsplätze der öffentlichen Dienstleistungen durch die
    % gesamten Erwerbstätigen geteilt werden und als Ausgleichfaktor mit drei
    % multipliziert wird. Somit ist es optimal wenn min. 1/3 aller
    % Erwerbsfähigen bei den öffentlichen Dienstleistungen arbeiten
    Dienstleistungsqualitaet = max(0.2, min(1, 3 * Arbeitsplaetze / Erwerbsfaehige));

== matlab function Waehrungsmodelle/Freies Geld Währungssystem/Notenbank/MATLAB Function ==
  data: Gesamtkredite input; LeitzinsOut output; MindestreservesatzOut output; MaximaleNotenbankGeldmengeOut output; Arbeitslosenquote input; Inflation input; Wirtschaftswachtsum input
function [LeitzinsOut, MindestreservesatzOut, MaximaleNotenbankGeldmengeOut] = ...
    Notenbank(Gesamtkredite, Arbeitslosenquote, Inflation, Wirtschaftswachtsum)
%# Submodul zur Berechnung der Notenbankprozesse

% Leitzins der Notenbank => 0.03
persistent Leitzins;

% Mindestreservesatz => 0.01
persistent Mindestreservesatz;    

% Maximale Geldmenge, welche von der Notenbank vergeben werden kann
persistent MaximaleNotenbankGeldmenge;   

% festgelegter Geldmengenwachstum => 0.05
% Dieser Wert ist bei gedeckten Währungssystemen notwendig, da hiermit die
% Geldmenge mit dem Gesamtwert des Deckungswerts mitwachsen kann
Geldmengenwachstum = 0.05;

% gewünschte Inflation => 0.02
Inflationsziel = 0.02;

% Inflationstoleranz => 0.02
Inflationstoleranz = 0.02;

% Arbeitslosentoleranzquote => 0.08
Arbeitslosentoleranzquote = 0.08;

% Änderung des Leitzins
Leitzinsaenderung = 0;

    if isempty(Leitzins)
       Leitzins = 0.03;
    end  
    if isempty(Mindestreservesatz)
       Mindestreservesatz = 0.01;
    end  
    if isempty(MaximaleNotenbankGeldmenge)
       MaximaleNotenbankGeldmenge =  1000;
    end       
    
    % Pürfen, ob ein erlaubter Geldmengenwachstum sinnvoll ist
    if Gesamtkredite > MaximaleNotenbankGeldmenge * 0.9
        MaximaleNotenbankGeldmenge = MaximaleNotenbankGeldmenge * (1 + Geldmengenwachstum);
    end
    
    % Wenn das Wirtschaftswachtsum zu gering ist, wird der Leitzins gesenkt
    if Wirtschaftswachtsum < Leitzins
        Leitzinsaenderung = -0.001;
    else
        Leitzinsaenderung = 0.001;
    end
    
    % Wenn die Arbeitslosigkeit unter der Arbeitslosentoleranzquote ist, wird kann der Leitzins erhöht
    % sonst wird der Leitzins in Abhängigkeit der Arbeitslosenquote gesenkt
    Leitzinsaenderung = Leitzinsaenderung + max(-0.01,0.1 * (Arbeitslosentoleranzquote - Arbeitslosenquote) + 0.001); 
    
    % Inflation mit dem Leitzins an die Zielinflation anpassen
    Leitzinsaenderung = Leitzinsaenderung + 0.01 * (Inflation - (Inflationsziel + Inflationstoleranz));
        
    if Leitzins < 0.01 && Leitzinsaenderung < -0.001
        Leitzins = Leitzins - 0.001;
    else        
        Leitzins = Leitzins + Leitzinsaenderung;
    end       
        
    
LeitzinsOut = Leitzins;
MindestreservesatzOut = Mindestreservesatz;
MaximaleNotenbankGeldmengeOut = MaximaleNotenbankGeldmenge;
